simulink model "gncTaira307"  (R2024b)
settings: Solver=VariableStepAuto  StartTime=0.0  StopTime=TF  RelTol=1e-3
values from neighbouring files (symbols this model uses):
  u1max = 25 * pi/180    (= 0.436332312999)    [initConstants.m]
  u1min = -25 * pi/180    (= -0.436332312999)    [initConstants.m]
  u2max = 10 * pi/180    (= 0.174532925199)    [initConstants.m]
  u2min = -25 * pi/180    (= -0.436332312999)    [initConstants.m]
  u3max = 30 * pi/180    (= 0.523598775598)    [initConstants.m]
  u3min = -30 * pi/180    (= -0.523598775598)    [initConstants.m]
  u4max = 10 * pi/180    (= 0.174532925199)    [initConstants.m]
  u4min = 0.5 * pi/180    (= 0.00872664625997)    [initConstants.m]
  u5max = 10 * pi/180    (= 0.174532925199)    [initConstants.m]
  u5min = 0.5 * pi/180    (= 0.00872664625997)    [initConstants.m]
  x0 = [85 ... (first row only)    [initConstants.m]
undefined symbols (not defined in the file or in its folder): FixedWingPlaneModel
settings Model: Creator=mohammad.ghannam  LastModifiedBy=lahce

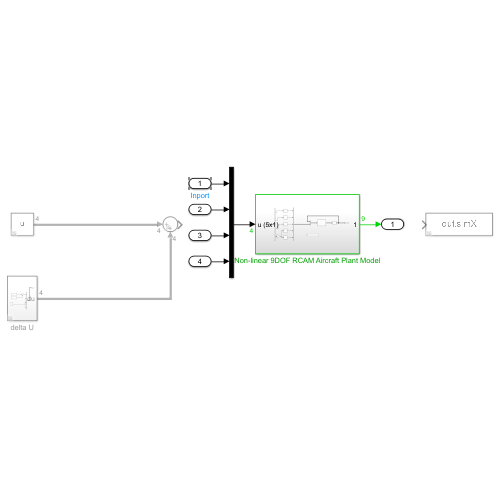
[thumbnail: Simulink's stored preview of the top-level diagram]
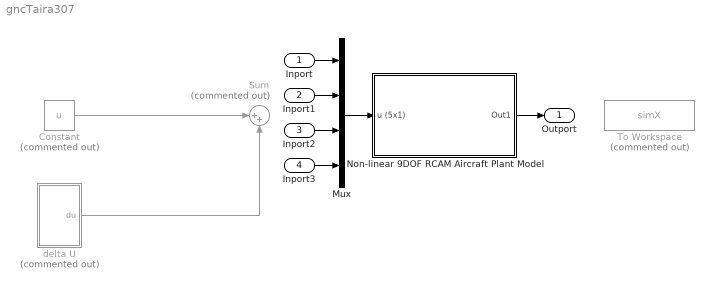
== system gncTaira307 ==
  Inport : Inport
  Inport1 : Inport  Port=2
  Inport2 : Inport  Port=3
  Inport3 : Inport  Port=4
  Constant : Constant  Commented=on  Value=u
  Mux : Mux
  Non-linear 9DOF RCAM Aircraft Plant Model : Subsystem
  Sum : Sum  Commented=on  Inputs=|++
  To Workspace : ToWorkspace  Commented=on  VariableName=simX  SaveFormat=Timeseries  SampleTime=-1
  delta U : Subsystem  Commented=on
  Outport : Outport
  wires:
  Constant/1 -> Sum/1
  delta U/1(du) -> Sum/2
  Inport1/1 -> Mux/2
  Inport3/1 -> Mux/4
  Mux/1 -> Non-linear 9DOF RCAM Aircraft Plant Model/1(u (5x1))
  Inport2/1 -> Mux/3
  Inport/1 -> Mux/1
  Non-linear 9DOF RCAM Aircraft Plant Model/1(Out1) -> Outport/1

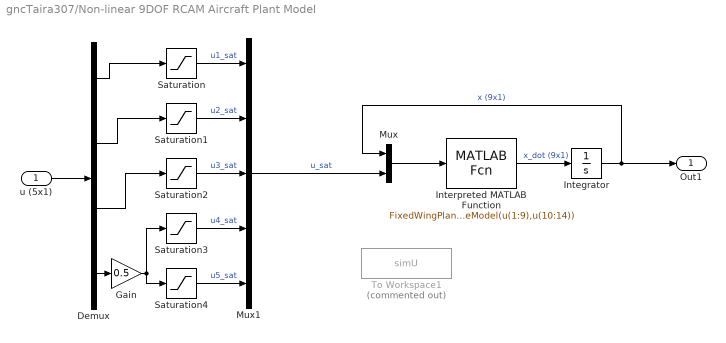
== system gncTaira307/Non-linear 9DOF RCAM Aircraft Plant Model ==
  u (5x1) : Inport
  Demux : Demux
  Gain : Gain  Gain=0.5
  Integrator : Integrator  InitialCondition=x0
  Interpreted MATLAB Function : MATLABFcn  MATLABFcn=FixedWingPlaneModel(u(1:9),u(10:14))
  Mux : Mux  Inputs=2
  Mux1 : Mux  Inputs=5
  Saturation : Saturate  UpperLimit=u1max  LowerLimit=u1min
  Saturation1 : Saturate  UpperLimit=u2max  LowerLimit=u2min
  Saturation2 : Saturate  UpperLimit=u3max  LowerLimit=u3min
  Saturation3 : Saturate  UpperLimit=u4max  LowerLimit=u4min
  Saturation4 : Saturate  UpperLimit=u5max  LowerLimit=u5min
  To Workspace1 : ToWorkspace  Commented=on  VariableName=simU  SaveFormat=Timeseries  SampleTime=-1
  Out1 : Outport
  wires:
  Integrator/1 -> Out1/1, Mux/1  "x (9x1)"
  Mux/1 -> Interpreted MATLAB Function/1
  Interpreted MATLAB Function/1 -> Integrator/1  "x_dot (9x1)"
  Demux/2 -> Saturation1/1
  u (5x1)/1 -> Demux/1
  Demux/1 -> Saturation/1
  Demux/3 -> Saturation2/1
  Saturation/1 -> Mux1/1  "u1_sat"
  Saturation1/1 -> Mux1/2  "u2_sat"
  Saturation2/1 -> Mux1/3  "u3_sat"
  Saturation3/1 -> Mux1/4  "u4_sat"
  Saturation4/1 -> Mux1/5  "u5_sat"
  Mux1/1 -> Mux/2  "u_sat"
  Demux/4 -> Gain/1
  Gain/1 -> Saturation4/1, Saturation3/1

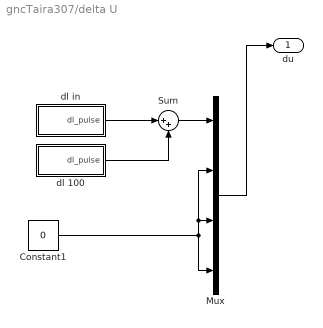
== system gncTaira307/delta U ==
  Constant1 : Constant  Value=0
  Mux : Mux
  Sum : Sum  Inputs=|++
  dl 100 : Subsystem
  dl in : Subsystem
  du : Outport
  wires:
  Constant1/1 -> Mux/2, Mux/3, Mux/4
  Mux/1 -> du/1
  Sum/1 -> Mux/1
  dl in/1(dl_pulse) -> Sum/1
  dl 100/1(dl_pulse) -> Sum/2

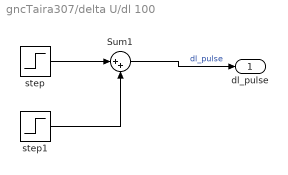
== system gncTaira307/delta U/dl 100 ==
  Sum1 : Sum  Inputs=|++
  step : Step  Time=100  After=-5 * pi/180  SampleTime=0
  step1 : Step  Time=102  After=5 * pi/180  SampleTime=0
  dl_pulse : Outport
  wires:
  Sum1/1 -> dl_pulse/1  "dl_pulse"
  step/1 -> Sum1/1
  step1/1 -> Sum1/2

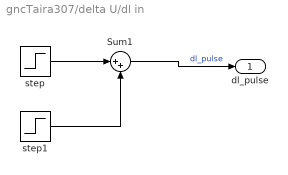
== system gncTaira307/delta U/dl in ==
  Sum1 : Sum  Inputs=|++
  step : Step  Time=30  After=5 * pi/180  SampleTime=0
  step1 : Step  Time=32  After=-5 * pi/180  SampleTime=0
  dl_pulse : Outport
  wires:
  Sum1/1 -> dl_pulse/1  "dl_pulse"
  step/1 -> Sum1/1
  step1/1 -> Sum1/2
